simulink model "Model_40_01_3"  (R2024b)
settings: Solver=VariableStepAuto  StartTime=0.0  StopTime=50  RelTol=1e-3
undefined symbols (not defined in the file): Atot, K, lab1P, z0_aug
settings Model: Creator=eddyp  LastModifiedBy=ricki

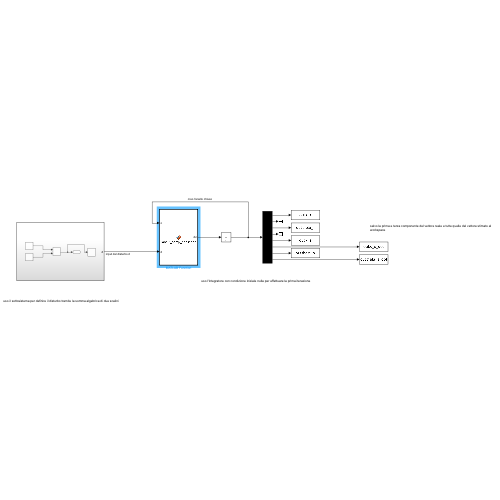
[thumbnail: Simulink's stored preview of the top-level diagram]
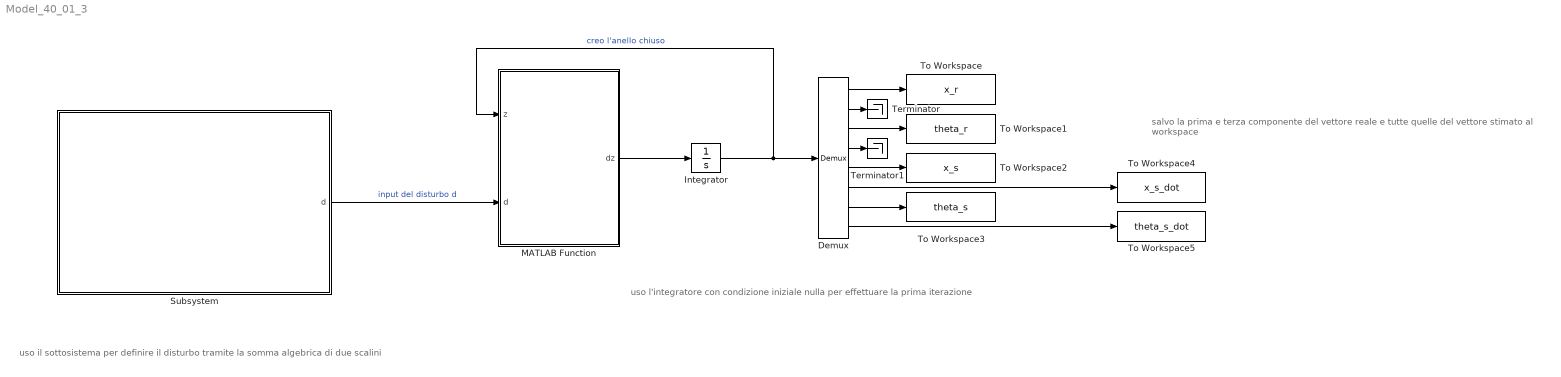
== system Model_40_01_3 ==
  note: uso l'integratore con condizione iniziale nulla per effettuare la prima iterazione
  note: uso il sottosistema per definire il disturbo tramite la somma algebrica di due scalini
  note: salvo la prima e terza componente del vettore reale e tutte quelle del vettore stimato al workspace
  Demux : Demux  Outputs=8
  Integrator : Integrator  InitialCondition=z0_aug
  MATLAB Function : MATLAB Function  TreatAsAtomicUnit=on
  Subsystem : Subsystem
  Terminator : Terminator
  Terminator1 : Terminator
  To Workspace : ToWorkspace  VariableName=x_r  SampleTime=-1
  To Workspace1 : ToWorkspace  VariableName=theta_r  SampleTime=-1
  To Workspace2 : ToWorkspace  VariableName=x_s  SampleTime=-1
  To Workspace3 : ToWorkspace  VariableName=theta_s  SampleTime=-1
  To Workspace4 : ToWorkspace  VariableName=x_s_dot  SampleTime=-1
  To Workspace5 : ToWorkspace  VariableName=theta_s_dot  SampleTime=-1
  wires:
  Subsystem/1(d) -> MATLAB Function/2(d)  "input del disturbo d"
  MATLAB Function/1(dz) -> Integrator/1
  Integrator/1 -> Demux/1, MATLAB Function/1(z)  "creo l'anello chiuso"
  Demux/8 -> To Workspace5/1
  Demux/1 -> To Workspace/1
  Demux/3 -> To Workspace1/1
  Demux/2 -> Terminator/1
  Demux/4 -> Terminator1/1
  Demux/5 -> To Workspace2/1
  Demux/7 -> To Workspace3/1
  Demux/6 -> To Workspace4/1

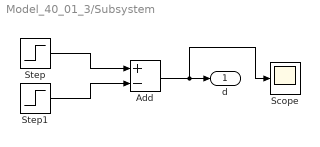
== system Model_40_01_3/Subsystem ==
  Add : Sum  Inputs=+-
  Scope : Scope
  Step : Step  SampleTime=0
  Step1 : Step  Time=3  SampleTime=0
  d : Outport
  wires:
  Step/1 -> Add/1
  Step1/1 -> Add/2
  Add/1 -> Scope/1, d/1

== matlab function Model_40_01_3/MATLAB Function ==
  data: dz output double size=[8,1]; z input size=[8,1]; d input; Atot parameter; K parameter; lab1P parameter
function dz = lab1P_comp_nonlinear( z, d,Atot,K, lab1P)
% la funzione riceve come input z e d, come parametri Atot e K. Restituisce
% come output il risultato dz, costituito da dz real e dz stimato. 
    % z è il vettore di stato aumentato 8x1:
    % z(1:4) è lo stato reale 
    % z(5:8) è lo stato stimato 
    
   
Atot = real(Atot); % rendo la matrice A del sistema aumentato appartenente ai numeri reali per evitare problemi di calcolo complesso
K = real(K);  % rendo la matrice dei guadagni del sistema aumentato appartenente ai numeri reali per evitare problemi di calcolo complesso
dz = zeros(8, 1);% inizializzo a zero il risultato
     
    % Il controllore calcola la corrente con la stima dell'osservatore (stati da 5 a 8).
    ii = - K * z(5:8);

   
    den = (lab1P.I0*lab1P.I2 - lab1P.I1^2*cos(z(3))^2 + lab1P.I2*lab1P.M);
    
    dz_reale = [
        z(2);
        
        -(- lab1P.g*sin(z(3))*lab1P.I1^2*cos(z(3)) + lab1P.I2*sin(z(3))*lab1P.I1*z(4)^2 + lab1P.b*lab1P.I1*z(4)*cos(z(3)) - lab1P.alpha1*d*lab1P.I1*cos(z(3))^2 + lab1P.I2*lab1P.alpha0*d - lab1P.I2*lab1P.alpham*ii + lab1P.I2*lab1P.c*z(2))/den;
        
        z(4);
        
        -(lab1P.I0*lab1P.b*z(4) + lab1P.M*lab1P.b*z(4) - lab1P.I0*lab1P.I1*lab1P.g*sin(z(3)) - lab1P.I1*lab1P.M*lab1P.g*sin(z(3)) - lab1P.I0*lab1P.alpha1*d*cos(z(3)) + lab1P.I1*lab1P.alpha0*d*cos(z(3)) - lab1P.M*lab1P.alpha1*d*cos(z(3)) - lab1P.I1*lab1P.alpham*ii*cos(z(3)) + lab1P.I1*lab1P.c*z(2)*cos(z(3)) + lab1P.I1^2*z(4)^2*cos(z(3))*sin(z(3)))/den
    ];

   
    dz_stimato = Atot(5:8, :) * z;

   
   dz(1:4) = dz_reale;
    dz(5:8) = dz_stimato; % ottengo dz concatenando i vettori reali e stimato
end
